simulink model "uav_simulation_tarotold"  (R2020a)
settings: Solver=VariableStepAuto  StartTime=0.0  StopTime=sim_params.max_sim_time  RelTol=1e-3
undefined symbols (not defined in the file): deg, DiscIntNeverNeededParam, F, Light, MIL, processes, rad, s, sim_params, trajectory, uav
libraries: aerolibconvert2 x2, dspstat3 x2, shared6dof x1, aerolibwind2 x1, sharedTrackingLibrary x1
(part 2 of 2)

== system uav_simulation_tarotold/Motors/DC Motor 6/Mechanical part ==
  Static Friction Torque : Inport
  Electrical Torque : Inport  Port=2
  1/J Inertia constant : Gain  Gain=1/uav.motors(6).J
  "Df viscous damping coefficient Dynamic Friction coefficient " : Gain  Gain=uav.motors(6).Df
  Discrete-Time Integrator : DiscreteIntegrator  gainval=1  InitialCondition=sim_params.initial_conditions.w6  SampleTime=uav.dynamics_srate  ICPrevOutput=DiscIntNeverNeededParam  ICPrevScaledInput=DiscIntNeverNeededParam
  Gain : Gain  Gain=uav.motors(6).cq
  Square : Math  Operator=square  SaturateOnIntegerOverflow=on
  Sum1 : Sum  Inputs=--+-
  w angular speed : Outport  VectorParamsAs1DForOutWhenUnconnected=off
  Torque : Outport  Port=2  VectorParamsAs1DForOutWhenUnconnected=off
  wires:
  1/J Inertia constant/1 -> Discrete-Time Integrator/1
  Static Friction Torque/1 -> Sum1/2
  "Df viscous damping coefficient Dynamic Friction coefficient "/1 -> Sum1/4
  Discrete-Time Integrator/1 -> w angular speed/1, Square/1, "Df viscous damping coefficient Dynamic Friction coefficient "/1  "w angular speed"
  Sum1/1 -> 1/J Inertia constant/1
  Electrical Torque/1 -> Sum1/3
  Gain/1 -> Torque/1, Sum1/1
  Square/1 -> Gain/1

== system uav_simulation_tarotold/Motors/DC Motor 7/Electrical part ==
  ESC voltage : Inport
  w angular speed : Inport  Port=2
  1/R : Gain  Gain=1/uav.motors(7).Req
  Ke (Torque constant)1 : Gain  Gain=uav.motors(7).Ke_eq
  Kt (Torque constant) Kt=Ke for an ideal square wave motor : Gain  Gain=uav.motors(7).Ke_eq
  Saturation : Saturate  UpperLimit=11  LowerLimit=0
  Sum : Sum  Inputs=|+-
  Electrical Torque : Outport  VectorParamsAs1DForOutWhenUnconnected=off
  current : Outport  Port=2  VectorParamsAs1DForOutWhenUnconnected=off
  wires:
  1/R/1 -> Saturation/1  "current i"
  Sum/1 -> 1/R/1
  Kt (Torque constant) Kt=Ke for an ideal square wave motor/1 -> Electrical Torque/1
  Ke (Torque constant)1/1 -> Sum/2
  ESC voltage/1 -> Sum/1
  w angular speed/1 -> Ke (Torque constant)1/1
  Saturation/1 -> Kt (Torque constant) Kt=Ke for an ideal square wave motor/1, current/1

== system uav_simulation_tarotold/Motors/DC Motor 7/Mechanical part ==
  Static Friction Torque : Inport
  Electrical Torque : Inport  Port=2
  1/J Inertia constant : Gain  Gain=1/uav.motors(7).J
  "Df viscous damping coefficient Dynamic Friction coefficient " : Gain  Gain=uav.motors(7).Df
  Discrete-Time Integrator : DiscreteIntegrator  gainval=1  InitialCondition=sim_params.initial_conditions.w7  SampleTime=uav.dynamics_srate  ICPrevOutput=DiscIntNeverNeededParam  ICPrevScaledInput=DiscIntNeverNeededParam
  Gain : Gain  Gain=uav.motors(7).cq
  Square : Math  Operator=square  SaturateOnIntegerOverflow=on
  Sum1 : Sum  Inputs=--+-
  w angular speed : Outport  VectorParamsAs1DForOutWhenUnconnected=off
  Torque : Outport  Port=2  VectorParamsAs1DForOutWhenUnconnected=off
  wires:
  1/J Inertia constant/1 -> Discrete-Time Integrator/1
  Static Friction Torque/1 -> Sum1/2
  "Df viscous damping coefficient Dynamic Friction coefficient "/1 -> Sum1/4
  Discrete-Time Integrator/1 -> w angular speed/1, Square/1, "Df viscous damping coefficient Dynamic Friction coefficient "/1  "w angular speed"
  Sum1/1 -> 1/J Inertia constant/1
  Electrical Torque/1 -> Sum1/3
  Gain/1 -> Torque/1, Sum1/1
  Square/1 -> Gain/1

== system uav_simulation_tarotold/Motors/DC Motor 8/Electrical part ==
  ESC voltage : Inport
  w angular speed : Inport  Port=2
  1/R : Gain  Gain=1/uav.motors(8).Req
  Ke (Torque constant)1 : Gain  Gain=uav.motors(8).Ke_eq
  Kt (Torque constant) Kt=Ke for an ideal square wave motor : Gain  Gain=uav.motors(8).Ke_eq
  Saturation : Saturate  UpperLimit=11  LowerLimit=0
  Sum : Sum  Inputs=|+-
  Electrical Torque : Outport  VectorParamsAs1DForOutWhenUnconnected=off
  current : Outport  Port=2  VectorParamsAs1DForOutWhenUnconnected=off
  wires:
  1/R/1 -> Saturation/1  "current i"
  Sum/1 -> 1/R/1
  Kt (Torque constant) Kt=Ke for an ideal square wave motor/1 -> Electrical Torque/1
  Ke (Torque constant)1/1 -> Sum/2
  ESC voltage/1 -> Sum/1
  w angular speed/1 -> Ke (Torque constant)1/1
  Saturation/1 -> Kt (Torque constant) Kt=Ke for an ideal square wave motor/1, current/1

== system uav_simulation_tarotold/Motors/DC Motor 8/Mechanical part ==
  Static Friction Torque : Inport
  Electrical Torque : Inport  Port=2
  1/J Inertia constant : Gain  Gain=1/uav.motors(8).J
  "Df viscous damping coefficient Dynamic Friction coefficient " : Gain  Gain=uav.motors(8).Df
  Discrete-Time Integrator : DiscreteIntegrator  gainval=1  InitialCondition=sim_params.initial_conditions.w8  SampleTime=uav.dynamics_srate  ICPrevOutput=DiscIntNeverNeededParam  ICPrevScaledInput=DiscIntNeverNeededParam
  Gain : Gain  Gain=uav.motors(8).cq
  Square : Math  Operator=square  SaturateOnIntegerOverflow=on
  Sum1 : Sum  Inputs=--+-
  w angular speed : Outport  VectorParamsAs1DForOutWhenUnconnected=off
  Torque : Outport  Port=2  VectorParamsAs1DForOutWhenUnconnected=off
  wires:
  1/J Inertia constant/1 -> Discrete-Time Integrator/1
  Static Friction Torque/1 -> Sum1/2
  "Df viscous damping coefficient Dynamic Friction coefficient "/1 -> Sum1/4
  Discrete-Time Integrator/1 -> w angular speed/1, Square/1, "Df viscous damping coefficient Dynamic Friction coefficient "/1  "w angular speed"
  Sum1/1 -> 1/J Inertia constant/1
  Electrical Torque/1 -> Sum1/3
  Gain/1 -> Torque/1, Sum1/1
  Square/1 -> Gain/1

== matlab function uav_simulation_tarotold/Motors/DC Motor 2/Simulink Function/MATLAB Function ==
  data: x input; u input; x output; param input
function x = MotorMeasurementFcn(x,u,param)

x = double(x*u(2) + param*u(1));

end

== matlab function uav_simulation_tarotold/Adding noise ==
  data: u input; y output; t input
function y = fcn(u,t)
if t==2.99
    see=1;
end
y = zeros(6,1);
% posnoisestd=0.75; % gives maximum and minimum of +-3 meters
posnoisestd=0.1; % gives maximum and minimum of +-.5 meters
velnoisestd=0.005;
noisepos=posnoisestd.*randn(3,1);
noisevel=velnoisestd.*randn(3,1);
noise=[noisepos ;noisevel];
y = y + u + noise;

== matlab function uav_simulation_tarotold/Subsystem/MATLAB Function1 ==
  settings: updateMethod=DISCRETE  sampleTime=.2
  data: mu input; y output; sigma input
function y = addNoise(mu, sigma)

y = normrnd(mu, sigma);

== matlab function uav_simulation_tarotold/Forces and Moments Calculation ==
  data: w1 input; Fx output; w2 input; w3 input; w4 input; w5 input; w6 input; Fy output; Fz output; Mx output; My output; Mz output; w7 input; w8 input; Phi input; The input; Psi input; ct input; cq input; cq2 input; l input; m input
function [Fx,Fy,Fz,Mx,My,Mz] = fcn(w1,w2,w3,w4,w5,w6,w7,w8,Phi,The,Psi, ct, cq, cq2, l, m)
g=9.80;

% Phi,The,Psi, in rad
w  = [w1; w2; w3; w4;w5; w6; w7; w8];

%% not used
%to fix numerical issues
%w=round(w,2);
% transform rpm to rad/s
%w=w./(60/(2*pi));

%thrust = ct * density of air * velocity^2 * propeller diameter (m) ^4
%velocity in rev/sec, where  1 rev/sec = 1 rpm/60
T = ct*1.225*((w./60).^2)*.47^4; % 18.5 inches ~ 0.47 m
% total thrust generated by rotors
T_total=sum(T);
T_total=round(T_total*100)/100;

%% Forces in the local frame 
R_b_e = [cos(Psi)*cos(The) cos(Psi)*sin(The)*sin(Phi)-sin(Psi)*cos(Phi) cos(Psi)*sin(The)*cos(Phi)+sin(Psi)*sin(Phi);
       sin(Psi)*cos(The) sin(Psi)*sin(The)*sin(Phi)+cos(Psi)*cos(Phi) sin(Psi)*sin(The)*cos(Phi)-cos(Psi)*sin(Phi);
       -sin(The)         cos(The)*sin(Phi)                            cos(The)*cos(Phi)]; % Rib

Ftot_b=R_b_e'*[0 ;0; -m*g]+[0; 0; T_total]; 
Fx=Ftot_b(1);Fy=Ftot_b(2);Fz=Ftot_b(3);

%% Moments in the local frame 
% moment of each rotor
M = (cq)*w.^2 + (cq2)*w ;

% torque generated by rotors
Mx=l*(T(1)+ (sqrt(2)/2)*T(2)+ (sqrt(2)/2)*T(8) ...
    - T(5)- (sqrt(2)/2)*T(4)- (sqrt(2)/2)*T(6));%Tau_roll

My=l*(T(7)+ (sqrt(2)/2)*T(6)+ (sqrt(2)/2)*T(8) ...
    - T(3)- (sqrt(2)/2)*T(2)- (sqrt(2)/2)*T(4));%Tau_theta

Mz= -M(1) +M(2) -M(3) +M(4) -M(5) +M(6) -M(7) +M(8);%%Tau_yaw
end

== matlab function uav_simulation_tarotold/arrival condition ==
  data: currentpos input; arrived output; dest input
function arrived = fcn(currentpos,dest)

result=norm(currentpos-dest);
if result<1 % less than one meter from the goal
    arrived=1;
else
    arrived=0;
end

== matlab function uav_simulation_tarotold/Motors/DC Motor 2/MATLAB Function ==
  settings: updateMethod=DISCRETE  sampleTime=.2
  data: mu input; y output; sigma input
function y = addNoise(mu, sigma)

y = normrnd(mu, sigma);

== matlab function uav_simulation_tarotold/Motors/DC Motor 2/MATLAB Function1 ==
  settings: updateMethod=DISCRETE  sampleTime=.2
  data: mu input; y output; sigma input
function y = addNoise(mu, sigma)

y = normrnd(mu, sigma);

== matlab function uav_simulation_tarotold/Control allocation ==
  data: Fx input; wref1 output; Fy input; Fz input; Troll input; Tpitch input; Tyaw input; wref2 output; wref3 output; wref4 output; wref5 output; wref6 output; wref7 output; wref8 output
function [wref1,wref2,wref3,wref4,wref5,wref6,wref7,wref8] = fcn(Fx,Fy,Fz,Troll,Tpitch,Tyaw)
%% parameters 
%Maximum speed that the motors can reach in rad/s, if I check voltage, I
%dont have to check speed
% Max_speed=710.31;
Max_speed=1000;

% arm length - distances from the octorotor center of mass ...
%        to the center of mass of all its rotors are equal and denoted by l.
l=0.35;
% thrust motor constant [Ns^2/rad^2]
b=8.54858e-06; % cq
% rotor drag constant [Nms^2/rad^2]
d=1.3678e-07; % ct
% control allocation matrix
A_f=[2*b 2*b 2*b 2*b; ...
    b*l 0 -b*l 0; ...
    -b*l -sqrt(2)*b*l b*l sqrt(2)*b*l; ...
    -2*d 2*d -2*d 2*d];
%desired input
u_des=[Fz;Troll;Tpitch;Tyaw];

%control allocation
Omega_sf=inv(A_f)*u_des;

%selection operator
E=[1 0 1 0 0 0 0 0;...
    0 1 0 1 0 0 0 0; ...
    0 0 0 0 1 0 1 0;...
    0 0 0 0 0 1 0 1]';

Omega_s=E*Omega_sf;

% velocity checking
wref=zeros(8);
for i=1:length(Omega_s)
    if Omega_s(i)<0
        wref(i)=0;
    elseif Omega_s(i)>Max_speed^2
        wref(i)=Max_speed;
    else
        wref(i)=sqrt(Omega_s(i));
    end
end

%velocity assignment in V
multiply=0.012240; %for 6783 rpm considering torque load 
for i=1:length(wref)
    % voltage saturation check
    if(wref(i)*multiply > 11.1)
        wref(i)=11.1;
    else
        wref(i)=wref(i)*multiply;
    end
end

wref1=wref(1);
wref2=wref(2);
wref3=wref(3);
wref4=wref(4);
wref5=wref(5);
wref6=wref(6);
wref7=wref(7);
wref8=wref(8);







% %% parameters required
% % load('params/octoModel.mat');
% gamma=3;%octomodel.tiltmotorangle;
% alpha=45;%octomodel.separationmotorangle;
% dl=0.45;%octomodel.dl;
% constant=(1/sqrt(2));
% ds=0.35;%octomodel.ds;
% ct=3.4262e-05;%octomodel.ct*(60/(2*pi))^2 -> in octomodel is for rpm, here I need it in rad/s;
% cq=9.3846e-07;%octomodel.cq*(60/(2*pi))^2 -> in octomodel is for rpm, here I need it in rad/s;
% 
% %% rotation matrices because of 3 degrees tilted angle
% 
% E_m_b = [0 -sin(alpha)*sin(gamma) sin(gamma) -cos(alpha)*sin(gamma) 0 sin(alpha)*sin(gamma) -sin(gamma) cos(alpha)*sin(gamma);
%          -sin(gamma)  cos(alpha)*sin(gamma) 0 -sin(alpha)*sin(gamma) sin(gamma) -cos(alpha)*sin(gamma) 0 sin(alpha)*sin(gamma);
%          -cos(gamma) -cos(gamma) -cos(gamma) -cos(gamma) -cos(gamma) -cos(gamma) -cos(gamma) -cos(gamma)];
% 
% R_m=[dl 0 0; ...
%     constant*ds constant*ds 0; ...
%     0 dl 0; ...
%     -constant*ds constant*ds 0; ...
%     -dl 0 0; ...
%     -constant*ds -constant*ds 0; ...
%     0 -dl 0; ...
%     constant*ds -constant*ds 0]';
% 
% %% first form delta_b matrix
% %a vectors
% a=zeros(3,8);
% for i=1:8
%     e_i_b=E_m_b(:,i);
%     a(:,i)=(ct).*e_i_b;
% end
% 
% %b vectors
% b=zeros(3,8);
% for i=1:8
%     e_i_b=E_m_b(:,i);
%     r_m=R_m(:,i);
%     b(:,i)=cross( r_m,(ct).*e_i_b ) + ((-1)^(i+1)*(cq)).*e_i_b;    
% end
% 
% %form matrix
% delta_b=[a;b];
% 
% %find pseudo-inverse
% delta_binv = pinv(delta_b);
% 
% %% calculate required w_ref
% Forces=[Fx,Fy,Fz];
% Torques=[Troll,Tpitch,Tyaw];
% if Troll>0
%     see=1;
% end
% input=[Forces,Torques]';
% wref=delta_binv*input;
% %check if complex
% if(isreal(wref(2)))
%     see=1;
% end
% 
% if length(find(wref<0))>0
%     pos=find(wref<0);
%     wref(pos)=0;
% end
% wref=sqrt(wref);
% 
% % %angular velocity in rad/s
% % wref1=wref(1);
% % wref2=wref(2);
% % wref3=wref(3);
% % wref4=wref(4);
% % wref5=wref(5);
% % wref6=wref(6);
% % wref7=wref(7);
% % wref8=wref(8);
% 
% %angular velocity in rpm
% % wref1=wref(1)*(60/(2*pi));
% % wref2=wref(2)*(60/(2*pi));
% % wref3=wref(3)*(60/(2*pi));
% % wref4=wref(4)*(60/(2*pi));
% % wref5=wref(5)*(60/(2*pi));
% % wref6=wref(6)*(60/(2*pi));
% % wref7=wref(7)*(60/(2*pi));
% % wref8=wref(8)*(60/(2*pi));
% 
% %% now convert to voltage in the range 0-22V
% % divide=36.17; %true is 36.37
% % multiply=0.0238; %for 8800 rpm nominal 
% multiply=0.02762; %for 6783 rpm considering torque load 
% wref1=wref(1)*multiply;
% wref2=wref(2)*multiply;
% wref3=wref(3)*multiply;
% wref4=wref(4)*multiply;
% wref5=wref(5)*multiply;
% wref6=wref(6)*multiply;
% wref7=wref(7)*multiply;
% wref8=wref(8)*multiply;
% 
% see=1;

end
